simulink library "Installation_Errors_Lib"  (R2023b)
settings: Solver=VariableStepAuto  StartTime=0.0  StopTime=10.0  RelTol=1e-3
undefined symbols (not defined in the file or in its folder): X_num
libraries: MISSILE_GUIDANCE_LIB2 x7, $bdroot x3, simulink x1
settings Model: Creator=leoni  LastModifiedBy=leoni

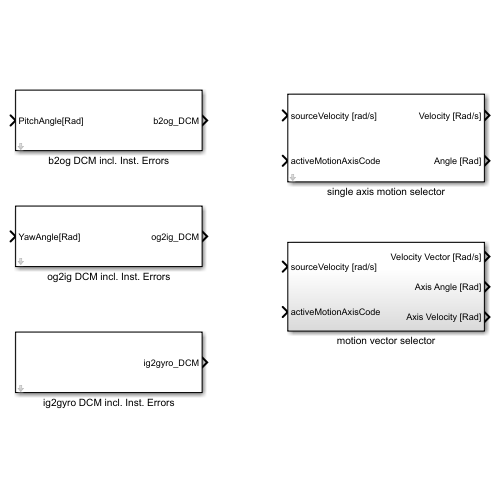
[thumbnail: Simulink's stored preview of the top-level diagram]
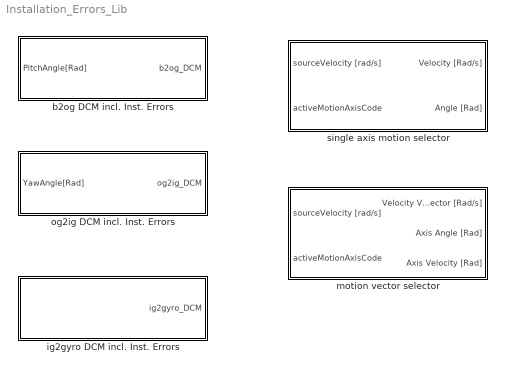
== system Installation_Errors_Lib ==
  b2og DCM incl. Inst. Errors : Subsystem  mask{eoa1=X_num(1), eoa3=X_num(2), theta_o=X_num(6)}
      mask prompts: eoa1 "eoa1[mRad]"; eoa3 "eoa3[mRad]"; theta_o "theta offset [mRad]"
      mask DialogControl ParameterGroupVar Prompt: Installation Errors
  ig2gyro DCM incl. Inst. Errors : Subsystem  mask{eg1=X_num(4), eg2=X_num(5)}
      mask prompts: eg1 "eg1 [mRad]"; eg2 "eg2 [mRad]"
      mask DialogControl ParameterGroupVar Prompt: Installation Errors
  motion vector selector : Subsystem
  og2ig DCM incl. Inst. Errors : Subsystem  mask{eia1=X_num(3), psi_o=X_num(7)}
      mask prompts: eia1 "eia1 [mRad]"; psi_o "psi offeset [mRad]"
      mask DialogControl ParameterGroupVar Prompt: Installation Errors
  single axis motion selector : Subsystem  mask{axisCode=Pitch}
      mask prompts: axisCode "What Axis it ?"

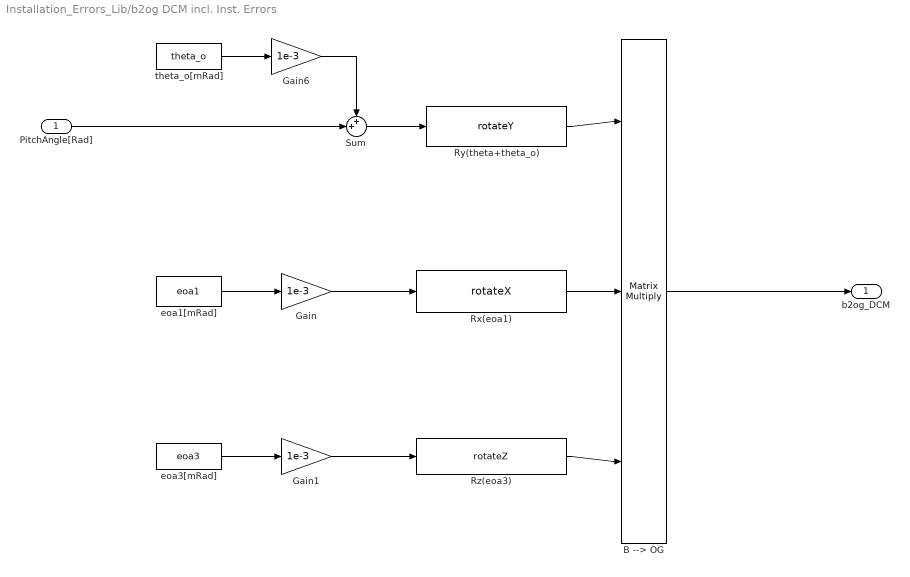
== system Installation_Errors_Lib/b2og DCM incl. Inst. Errors ==
  PitchAngle[Rad] : Inport
  B --> OG : Product  Inputs=3  Multiplication=Matrix(*)
  Gain : Gain  Gain=1e-3
  Gain1 : Gain  Gain=1e-3
  Gain6 : Gain  Gain=1e-3
  Rx(eoa1) : MISSILE_GUIDANCE_LIB2/rotateX  SystemSampleTime=-1  VariantActivationTime=update diagram  AllowFlexibleInterface=on  Latency=0  AutoFrameSizeCalculation=off
  Ry(theta+theta_o) : MISSILE_GUIDANCE_LIB2/rotateY  SystemSampleTime=-1  VariantActivationTime=update diagram  AllowFlexibleInterface=on  Latency=0  AutoFrameSizeCalculation=off
  Rz(eoa3) : MISSILE_GUIDANCE_LIB2/rotateZ  SystemSampleTime=-1  VariantActivationTime=update diagram  AllowFlexibleInterface=on  Latency=0  AutoFrameSizeCalculation=off
  Sum : Sum  Inputs=++|
  eoa1[mRad] : Constant  Value=eoa1
  eoa3[mRad] : Constant  Value=eoa3
  theta_o[mRad] : Constant  Value=theta_o
  b2og_DCM : Outport
  wires:
  eoa1[mRad]/1 -> Gain/1
  B --> OG/1 -> b2og_DCM/1
  Rz(eoa3)/1 -> B --> OG/3
  Rx(eoa1)/1 -> B --> OG/2
  eoa3[mRad]/1 -> Gain1/1
  Gain/1 -> Rx(eoa1)/1
  Gain1/1 -> Rz(eoa3)/1
  Ry(theta+theta_o)/1 -> B --> OG/1
  PitchAngle[Rad]/1 -> Sum/2
  Gain6/1 -> Sum/1
  theta_o[mRad]/1 -> Gain6/1
  Sum/1 -> Ry(theta+theta_o)/1

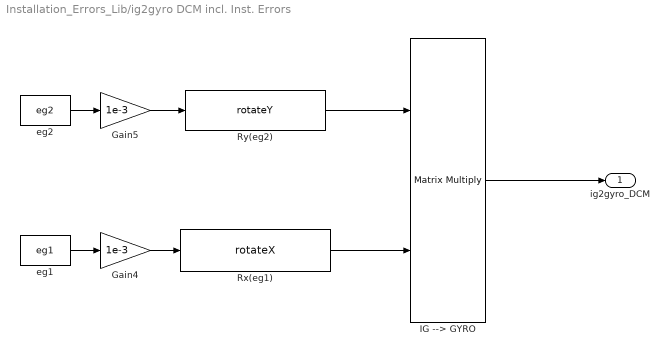
== system Installation_Errors_Lib/ig2gyro DCM incl. Inst. Errors ==
  Gain4 : Gain  Gain=1e-3
  Gain5 : Gain  Gain=1e-3
  IG --> GYRO : Product  Multiplication=Matrix(*)
  Rx(eg1) : MISSILE_GUIDANCE_LIB2/rotateX  SystemSampleTime=-1  VariantActivationTime=update diagram  AllowFlexibleInterface=on  Latency=0  AutoFrameSizeCalculation=off
  Ry(eg2) : MISSILE_GUIDANCE_LIB2/rotateY  SystemSampleTime=-1  VariantActivationTime=update diagram  AllowFlexibleInterface=on  Latency=0  AutoFrameSizeCalculation=off
  eg1 : Constant  Value=eg1
  eg2 : Constant  Value=eg2
  ig2gyro_DCM : Outport
  wires:
  IG --> GYRO/1 -> ig2gyro_DCM/1
  eg2/1 -> Gain5/1
  Gain4/1 -> Rx(eg1)/1
  eg1/1 -> Gain4/1
  Rx(eg1)/1 -> IG --> GYRO/2
  Gain5/1 -> Ry(eg2)/1
  Ry(eg2)/1 -> IG --> GYRO/1

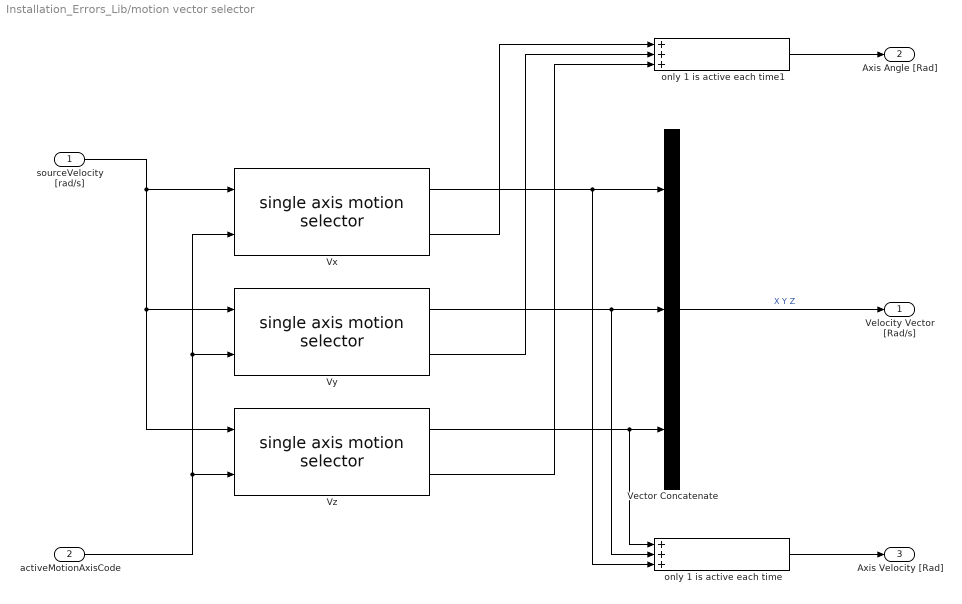
== system Installation_Errors_Lib/motion vector selector ==
  sourceVelocity [rad/s] : Inport
  activeMotionAxisCode : Inport  Port=2
  Vector Concatenate : Concatenate  NumInputs=3
  Vx : $bdroot/single axis motion selector  axisCode=Pitch
  Vy : $bdroot/single axis motion selector  axisCode=Pitch
  Vz : $bdroot/single axis motion selector  axisCode=Pitch
  only 1 is active each time : Sum  Inputs=+++
  only 1 is active each time1 : Sum  Inputs=+++
  Velocity Vector [Rad/s] : Outport
  Axis Angle [Rad] : Outport  Port=2
  Axis Velocity [Rad] : Outport  Port=3
  wires:
  activeMotionAxisCode/1 -> Vz/2, Vx/2, Vy/2
  sourceVelocity [rad/s]/1 -> Vz/1, Vy/1, Vx/1
  Vx/1 -> only 1 is active each time/3, Vector Concatenate/1
  Vy/1 -> only 1 is active each time/2, Vector Concatenate/2
  Vz/1 -> only 1 is active each time/1, Vector Concatenate/3
  Vector Concatenate/1 -> Velocity Vector [Rad/s]/1  "X Y Z"
  only 1 is active each time1/1 -> Axis Angle [Rad]/1
  only 1 is active each time/1 -> Axis Velocity [Rad]/1
  Vz/2 -> only 1 is active each time1/3
  Vy/2 -> only 1 is active each time1/2
  Vx/2 -> only 1 is active each time1/1

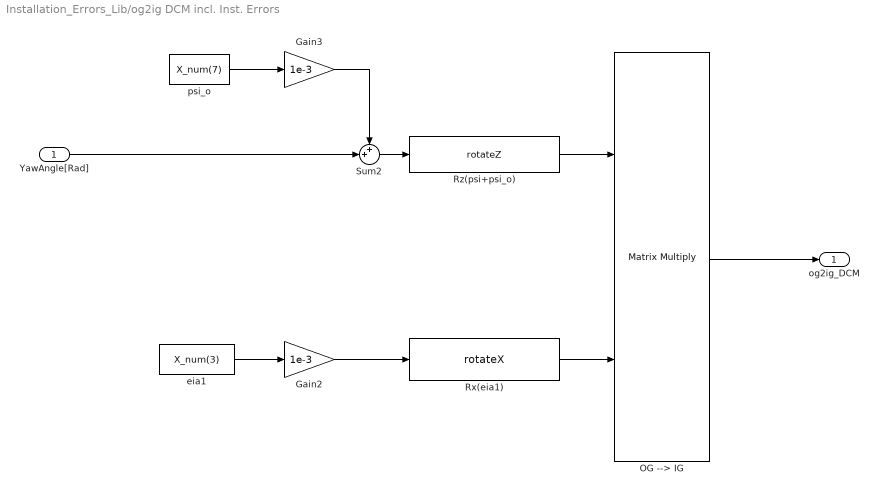
== system Installation_Errors_Lib/og2ig DCM incl. Inst. Errors ==
  "YawAngle[Rad] " : Inport
  Gain2 : Gain  Gain=1e-3
  Gain3 : Gain  Gain=1e-3
  OG --> IG : Product  Multiplication=Matrix(*)
  Rx(eia1) : MISSILE_GUIDANCE_LIB2/rotateX  SystemSampleTime=-1  VariantActivationTime=update diagram  AllowFlexibleInterface=on  Latency=0  AutoFrameSizeCalculation=off
  Rz(psi+psi_o) : MISSILE_GUIDANCE_LIB2/rotateZ  SystemSampleTime=-1  VariantActivationTime=update diagram  AllowFlexibleInterface=on  Latency=0  AutoFrameSizeCalculation=off
  Sum2 : Sum  Inputs=++|
  eia1 : Constant  Value=X_num(3)
  psi_o : Constant  Value=X_num(7)
  og2ig_DCM : Outport
  wires:
  Rx(eia1)/1 -> OG --> IG/2
  eia1/1 -> Gain2/1
  Gain2/1 -> Rx(eia1)/1
  Sum2/1 -> Rz(psi+psi_o)/1
  psi_o/1 -> Gain3/1
  Gain3/1 -> Sum2/1
  Rz(psi+psi_o)/1 -> OG --> IG/1
  "YawAngle[Rad] "/1 -> Sum2/2
  OG --> IG/1 -> og2ig_DCM/1

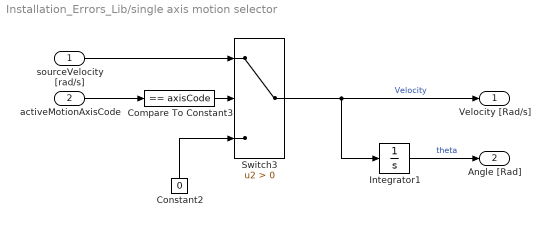
== system Installation_Errors_Lib/single axis motion selector ==
  sourceVelocity [rad/s] : Inport
  activeMotionAxisCode : Inport  Port=2
  Compare To Constant3 : simulink/Logic and Bit Operations/Compare To Constant  relop===  const=axisCode  OutDataTypeStr=boolean
  Constant2 : Constant  Value=0
  Integrator1 : Integrator
  Switch3 : Switch  Criteria=u2 > Threshold  SaturateOnIntegerOverflow=off  InputSameDT=off
  Velocity [Rad/s] : Outport
  Angle [Rad] : Outport  Port=2
  wires:
  sourceVelocity [rad/s]/1 -> Switch3/1
  Switch3/1 -> Integrator1/1, Velocity [Rad/s]/1  "Velocity"
  activeMotionAxisCode/1 -> Compare To Constant3/1
  Constant2/1 -> Switch3/3
  Compare To Constant3/1 -> Switch3/2
  Integrator1/1 -> Angle [Rad]/1  "theta"
